simulink library "bcm"  (R2021b)
settings: Solver=VariableStepAuto  StartTime=0.0  StopTime=10.0  RelTol=1e-3
undefined symbols (not defined in the file or in its folder): ENUM_ANTITHEFT_ALARM, ENUM_ANTITHEFT_ARM, ENUM_ANTITHEFT_DISARM, ENUM_ANTITHEFT_WAIT, ENUM_GEARPOSNTOCAN_P, ENUM_PDKEYRAWLULOCK_INUNLOCK, ENUM_PDKEYRAWPS_INPS, ENUM_POWERSTA_READY, ENUM_POWERSTA_STANDBY, FALSE, KBCM_ALMBrightnessDark_enum, KBCM_AmbBlue_enum, KBCM_AmbBreathT_K, KBCM_AmbBreathTOut_K, KBCM_AmbGreen_enum, KBCM_AmbLightUser_enum, KBCM_AmbPreset_enum, KBCM_AmbRed_enum, KBCM_Antitheft_enum_ovrdflg, KBCM_Antitheft_enum_ovrdval, KBCM_APMDoorCtrlSta_flg_ovrdflg, KBCM_APMDoorCtrlSta_flg_ovrdval, KBCM_DelayTSW_flg, KBCM_DiagFLTC_mA, KBCM_DiagFMHT_s, KBCM_DiagFRTC_mA, KBCM_DiagRLTC_mA, KBCM_DiagRRTC_mA, KBCM_DrAPMRetryTimes_cnt, KBCM_DrOpenWdwOT_s, KBCM_DrOpenWdwReady_s, KBCM_ESSOffT_ms, KBCM_ESSOnT_ms, KBCM_IVIRstHoldT_ms, KBCM_IVIRstTriggerT_ms, KBCM_ONDelayT_ms, KBCM_ReDetectT_K, KBCM_RmLampKeep_min, KBCM_RmLpKeyInT_s, KBCM_RmLpKeyMissT_s, KBCM_SlpDebounceTime_s, KBCM_SPTGDetectT_sec, KBCM_SPTGLeave_flg, KBCM_SPTGLeftBound_cm, KBCM_SPTGLeftBoundOut_cm, KBCM_SPTGLowerBound_cm, KBCM_SPTGLowerBoundOut_cm, KBCM_SPTGRightBound_cm, KBCM_SPTGRightBoundOut_cm, KBCM_SPTGTOut_K, KBCM_SPTGUpperBound_cm, KBCM_SPTGUpperBoundOut_cm, KBCM_SPTGWaitDKC_sec, KBCM_USSDis_cm, KBCM_USSFilterT_K, KBCM_WaitAPMPwr_K, KBCM_WdwManualDetT_s, MIN2SEC, TRUE, XX2KXX
libraries: simulink x41, $bdroot x3, hcu_lib x2
(part 5 of 6)

== stateflow chart bcm/BCM/BCM/ExteriorLight/Chart ==
  settings: updateMethod=DISCRETE
  state FollowMeSW [parallel]
    settings: executionOrder=2
    state sRelease
    state sPress
    (default) -> sRelease
    sRelease -> sPress : [VINP_FollowMeSW_flg==1]/{AutoCut.eFollow;}
    sPress -> sRelease : [VINP_FollowMeSW_flg==0]
  state RFogLamp [parallel]
    settings: executionOrder=1
    state sON
      en:VBCM_RrFogLamp_flg=1;
    state sOFF
      en:VBCM_RrFogLamp_flg=0;
    (default) -> RFogLamp.sOFF
    RFogLamp.sOFF -> RFogLamp.sON : [VPMM_PwrSta_enum>3&&....
        | VINP_RFogLampSW_flg==1&&....
        | VBCM_LBeam_flg==1]
    RFogLamp.sON -> RFogLamp.sOFF : [VPMM_PwrSta_enum<=3||....
        | VINP_RFogLampSW_flg==0||....
        | VBCM_LBeam_flg==0]
  state DRL [parallel]
    settings: executionOrder=3
    state sOFF
      en:VBCM_LDRL_flg=0;
      VBCM_RDRL_flg=0;
    state DRL_Opearting
      state sDebounce
      state sON
        en:VBCM_LDRL_flg=1;
        VBCM_RDRL_flg=1;
      note: 300 ms
      state TurnLeft
        en:VBCM_LDRL_flg=0;
        VBCM_RDRL_flg=1;
      state TurnRight
        en:VBCM_LDRL_flg=1;
        VBCM_RDRL_flg=0;
      sDebounce -> (junction 2687) : [after(30,tick)]
      (junction 2687) -> DRL.DRL_Opearting.sON [order 1] : [VBCM_OutMode_enum==0]
      (junction 2687) -> (junction 2689) [order 2]
      DRL.DRL_Opearting.sON -> TurnLeft [order 1] : [VBCM_OutMode_enum==1]
      TurnLeft -> DRL.DRL_Opearting.sON [order 1] : [VBCM_OutMode_enum==0]
      TurnRight -> DRL.DRL_Opearting.sON [order 2] : [VBCM_OutMode_enum==0]
      DRL.DRL_Opearting.sON -> TurnRight [order 2] : [VBCM_OutMode_enum==2]
      (junction 2689) -> TurnLeft [order 1] : [VBCM_OutMode_enum==1]
      (junction 2689) -> (junction 2701) [order 2]
      TurnRight -> TurnLeft [order 1] : [VBCM_OutMode_enum==1]
      TurnLeft -> TurnRight [order 2] : [VBCM_OutMode_enum==2]
      (junction 2701) -> TurnRight
    (default) -> DRL.sOFF
    DRL.sOFF -> sDebounce : [VBCM_DiagDRLOFF_flg==0 &&...
        | VPMM_PwrSta_enum==ENUM_POWERSTA_READY &&...
        | (VTQD_ShiftGearPosn_enum != ENUM_GEARPOSNTOCAN_P || VINP_HeadLampSW_enum==0) &&...
        | !VBCM_PosLamp_flg &&...
        | VBCM_OutMode_enum < 3]
    DRL_Opearting -> DRL.sOFF : [VBCM_DiagDRLOFF_flg==1 ||...
        | VPMM_PwrSta_enum!=ENUM_POWERSTA_READY ||...
        | (VTQD_ShiftGearPosn_enum == ENUM_GEARPOSNTOCAN_P && VINP_HeadLampSW_enum!=0) ||...
        | VBCM_PosLamp_flg ||...
        | VBCM_OutMode_enum >= 3]
  state sBrakeLamp [parallel]
    settings: executionOrder=4
    state sON
      en:VBCM_BrakeLamp_flg=1;
    state sOFF
      en:VBCM_BrakeLamp_flg=0;
    (default) -> sBrakeLamp.sOFF
    sBrakeLamp.sOFF -> sBrakeLamp.sON : [VINP_BrakeSWGPIO_flg==1 || VTQD_ReBrakeLPReq_flg==1 || VINP_ActBrkLampSta_flg==1]
    sBrakeLamp.sON -> sBrakeLamp.sOFF : [VINP_BrakeSWGPIO_flg==0 && VTQD_ReBrakeLPReq_flg==0 && VINP_ActBrkLampSta_flg==0]
  state sReverseLamp [parallel]
    settings: executionOrder=5
    state sON
      en:VBCM_ReverseLamp_flg=1;
    state sOFF
      en:VBCM_ReverseLamp_flg=0;
    (default) -> sReverseLamp.sOFF
    sReverseLamp.sOFF -> sReverseLamp.sON : [VPMM_PwrSta_enum>3&&VTQD_ShiftGearPosn_enum==7]
    sReverseLamp.sON -> sReverseLamp.sOFF : [VPMM_PwrSta_enum<=3||VTQD_ShiftGearPosn_enum!=7]
  state sATCtrl [parallel]
    settings: executionOrder=6
    state StandBy
    state Lock
      en:send(AutoCut.eLock);
    state Unlock
      en:send(AutoCut.eUnlock);
    (default) -> StandBy
    StandBy -> Lock [order 1] : [VBCM_ATCtrl_enum==1]
    Lock -> StandBy : [VBCM_ATCtrl_enum!=1]
    StandBy -> sATCtrl.Unlock [order 2] : [VBCM_ATCtrl_enum==2]
    sATCtrl.Unlock -> StandBy : [VBCM_ATCtrl_enum!=2]
  state PositionLamp [parallel]
    settings: executionOrder=11
    state sPositionLamp
      en:VBCM_PosLamp_flg=1;
    state sOFF
      en:VBCM_PosLamp_flg=0;
    (default) -> PositionLamp.sOFF
    (junction 2636) -> sPositionLamp [order 1] : [VINP_HeadLampSW_enum==1||VINP_HeadLampSW_enum==2]
    PositionLamp.sOFF -> (junction 2636) [order 1] : [!VBCM_AutoCut_flg]
    (junction 2636) -> (junction 2637) [order 2]
    (junction 2637) -> sPositionLamp [order 1] : [VPMM_PwrSta_enum>3&&VINP_HeadLampSW_enum==0&&VINP_RLSLampSta_flg]
    (junction 2637) -> (junction 2638) [order 2]
    (junction 2638) -> sPositionLamp : [VBCM_FollowMe_flg]
    PositionLamp.sOFF -> sPositionLamp [order 2] : [VBCM_showup_flg]
    (junction 2639) -> PositionLamp.sOFF : [!VBCM_FollowMe_flg&&(VINP_HeadLampSW_enum==3||....
        | (VINP_HeadLampSW_enum==0&&(VPMM_PwrSta_enum<=3||!VINP_RLSLampSta_flg)))]
    (junction 2640) -> (junction 2639) [order 2]
    (junction 2640) -> PositionLamp.sOFF [order 1] : [VBCM_AutoCut_flg]
    sPositionLamp -> (junction 2640) : [!VBCM_showup_flg]
  state AutoCut [parallel]
    settings: executionOrder=12
    state FollowMeHome
      en:
      VBCM_FollowMe_flg=1;
      VBCM_AutoCut_flg=0;
      VBCM_showup_flg=0;
      ex:
      VBCM_FollowMe_flg=0;
    state Normal
      state sNormal
        en:VBCM_AutoCut_flg=0;
        VBCM_showup_flg=0;
      state AutoCutDetect
      note: 40 sec
      state Unlock
        en:VBCM_AutoCut_flg=1;
        VBCM_showup_flg=1;
        note: 30 sec
      state AutoCut
        en:VBCM_AutoCut_flg=1;
        VBCM_showup_flg=0;
        VBCM_FollowMe_flg=0;
      sNormal -> AutoCutDetect : [VPMM_PwrSta_enum<=3&&(VINP_HeadLampSW_enum!=3)]
      (junction 2665) -> sNormal : [VPMM_PwrSta_enum>3||VINP_HeadLampSW_enum==3]
      AutoCutDetect -> (junction 2665) [order 1]
      AutoCut.Normal.AutoCut -> (junction 2665)
      AutoCutDetect -> AutoCut.Normal.AutoCut [order 2] : eLock
      AutoCutDetect -> AutoCut.Normal.AutoCut [order 3] : [after(4000,tick)]
      AutoCut.Normal.Unlock -> sNormal [order 2] : [VPMM_PwrSta_enum>3]
      (default) -> AutoCut.Normal.AutoCut
      AutoCut.Normal.Unlock -> AutoCut.Normal.AutoCut [order 1] : eLock
      AutoCut.Normal.Unlock -> AutoCut.Normal.AutoCut [order 3] : [after(3000,tick)]
      Normal -> AutoCut.Normal.Unlock [order 1] : eUnlock[VPMM_PwrSta_enum<=3]
    note: 4000
    note: 40 sec
    (default) -> Normal
    Normal -> FollowMeHome [order 1] : eFollow[VPMM_PwrSta_enum<=3]
    FollowMeHome -> sNormal [order 2] : eFollow
    FollowMeHome -> sNormal [order 3] : [VPMM_PwrSta_enum>3]
    FollowMeHome -> (junction 2717) [order 1] : [after(VBCM_DiagFMHT_s,tick)]
    (junction 2717) -> sNormal [order 1] : [VPMM_PwrSta_enum>3||...
        |  VINP_HeadLampSW_enum==3]
    (junction 2717) -> (junction 2719) [order 2]
    (junction 2719) -> AutoCut.Normal.AutoCut
  state LowBeam [parallel]
    settings: executionOrder=8
    state sLBeam
      en:VBCM_LBeam_flg=1;
    state sOFF
      en:VBCM_LBeam_flg=0;
    (default) -> LowBeam.sOFF
    (junction 2417) -> sLBeam [order 1] : [VBCM_HBeam_flg]
    LowBeam.sOFF -> (junction 2417) [order 1] : [!VBCM_AutoCut_flg]
    (junction 2417) -> (junction 2418) [order 2]
    (junction 2418) -> sLBeam [order 1] : [VINP_HeadLampSW_enum==2]
    (junction 2418) -> (junction 2419) [order 2]
    (junction 2419) -> sLBeam [order 1] : [VPMM_PwrSta_enum>3&&VINP_HeadLampSW_enum==0&&VINP_RLSLampSta_flg]
    (junction 2419) -> (junction 2420) [order 2]
    (junction 2420) -> sLBeam : [VBCM_FollowMe_flg]
    LowBeam.sOFF -> sLBeam [order 2] : [VBCM_showup_flg]
    (junction 2421) -> LowBeam.sOFF [order 1] : [VBCM_AutoCut_flg]
    sLBeam -> (junction 2421) : [!VBCM_showup_flg]
    (junction 2421) -> (junction 2422) [order 2]
    (junction 2422) -> LowBeam.sOFF : [!VBCM_FollowMe_flg&&!VBCM_HBeam_flg&&VINP_HeadLampSW_enum!=2&&....
        | (VINP_HeadLampSW_enum!=0||!VINP_RLSLampSta_flg||VPMM_PwrSta_enum<=3)]
  state HighBeam [parallel]
    settings: executionOrder=7
    state sHBeam
      en:VBCM_HBeam_flg=1;
    state sOFF
      en:VBCM_HBeam_flg=0;
    (default) -> HighBeam.sOFF
    HighBeam.sOFF -> (junction 2455) : [!VBCM_AutoCut_flg]
    (junction 2455) -> sHBeam [order 1] : [VINP_CSWPassSWSta_flg]
    (junction 2455) -> (junction 2456) [order 2]
    (junction 2456) -> (junction 2457) : [VINP_CSWDimSw_flg]
    (junction 2457) -> sHBeam [order 1] : [VINP_HeadLampSW_enum==2]
    (junction 2457) -> (junction 2458) [order 2]
    (junction 2458) -> sHBeam : [VINP_HeadLampSW_enum==0&&VINP_RLSLampSta_flg==1&&VINP_ForceLowBeam_enum==0&&VPMM_PwrSta_enum>3&&VBCM_AutoHLB_flg]
    sHBeam -> HighBeam.sOFF [order 1] : [VBCM_AutoCut_flg]
    (junction 2459) -> HighBeam.sOFF [order 1] : [!VINP_CSWDimSw_flg]
    sHBeam -> (junction 2459) [order 2] : [!VINP_CSWPassSWSta_flg]
    (junction 2459) -> (junction 2605) [order 2]
    (junction 2460) -> HighBeam.sOFF [order 1] : [VINP_HeadLampSW_enum!=0]
    (junction 2605) -> (junction 2460) : [VINP_HeadLampSW_enum!=2]
    (junction 2460) -> (junction 2462) [order 2]
    (junction 2462) -> HighBeam.sOFF [order 1] : [VINP_RLSLampSta_flg==0||VPMM_PwrSta_enum<=3]
    (junction 2462) -> (junction 2463) [order 2]
    (junction 2463) -> HighBeam.sOFF : [VINP_ForceLowBeam_enum==1||!VBCM_AutoHLB_flg]
  state AutoHLB [parallel]
    settings: executionOrder=13
    state AutoON
      on after(KBCM_ONDelayT_ms, tick):
      VBCM_AutoHLB_flg = TRUE;
    state AutoOFF
      en:
      VBCM_AutoHLB_flg = FALSE;
    (default) -> AutoOFF
    AutoOFF -> AutoON : [VINP_METERKPHCalcu_kph >= 30]
    AutoON -> AutoOFF : [VINP_METERKPHCalcu_kph <= 25]
  state RBSD_CTRL [parallel]
    settings: executionOrder=10
    state OFF
      en:VBCM_RBSD_flg=0;
    state FlashOFF
      en:VBCM_RBSD_flg=0;
    state ON
      en:VBCM_RBSD_flg=1;
    (default) -> RBSD_CTRL.OFF
    RBSD_CTRL.FlashOFF -> RBSD_CTRL.OFF [order 1] : [VINP_SRRBSDWarnR_flg==0 && VINP_SRRODAWarnR_flg==0]
    RBSD_CTRL.ON -> RBSD_CTRL.FlashOFF [order 2] : [after(13,tick)&&(VINP_SRRBSDWarnR_flg==2||VINP_SRRODAWarnR_flg==2)]
    RBSD_CTRL.FlashOFF -> RBSD_CTRL.ON [order 2] : [after(12,tick)]
    RBSD_CTRL.ON -> RBSD_CTRL.OFF [order 1] : [VINP_SRRBSDWarnR_flg==0 && VINP_SRRODAWarnR_flg==0]
    RBSD_CTRL.OFF -> RBSD_CTRL.ON : [VINP_SRRBSDWarnR_flg>0 || VINP_SRRODAWarnR_flg>0]
  state LBSD_CTRL [parallel]
    settings: executionOrder=9
    state OFF
      en:VBCM_LBSD_flg=0;
    state FlashOFF
      en:VBCM_LBSD_flg=0;
    state ON
      en:VBCM_LBSD_flg=1;
    (default) -> LBSD_CTRL.OFF
    LBSD_CTRL.FlashOFF -> LBSD_CTRL.OFF [order 1] : [VINP_SRRBSDWarnL_flg==0 && VINP_SRRODAWarnL_flg==0]
    LBSD_CTRL.ON -> LBSD_CTRL.FlashOFF [order 2] : [after(13,tick)&&(VINP_SRRBSDWarnL_flg==2||VINP_SRRODAWarnL_flg==2)]
    LBSD_CTRL.FlashOFF -> LBSD_CTRL.ON [order 2] : [after(12,tick)]
    LBSD_CTRL.ON -> LBSD_CTRL.OFF [order 1] : [VINP_SRRBSDWarnL_flg==0 && VINP_SRRODAWarnL_flg==0]
    LBSD_CTRL.OFF -> LBSD_CTRL.ON : [VINP_SRRBSDWarnL_flg>0 || VINP_SRRODAWarnL_flg>0]
  data: VPMM_PwrSta_enum input uint8 [0..5]; VINP_HeadLampSW_enum input uint8 [0..3]; VINP_RFogLampSW_flg input boolean; VINP_BrakeSWGPIO_flg input boolean; VINP_CSWDimSw_flg input boolean; VINP_CSWPassSWSta_flg input boolean; VTQD_ShiftGearPosn_enum input uint8 [0..15]; VBCM_PosLamp_flg output boolean; VBCM_LBeam_flg output boolean; VBCM_HBeam_flg output boolean; VBCM_RrFogLamp_flg output boolean; VBCM_BrakeLamp_flg output boolean; VBCM_ReverseLamp_flg output boolean; VBCM_OutMode_enum input uint8 [0..15]; VBCM_AutoCut_flg local boolean; VBCM_LDRL_flg output boolean; VBCM_RDRL_flg output boolean; VINP_FollowMeSW_flg input boolean; VBCM_ATCtrl_enum input uint8 [0..2]; VINP_RLSLampSta_flg input boolean; VINP_ActBrkLampSta_flg input boolean; VINP_SRRODAWarnR_flg input; VINP_SRRODAWarnL_flg input; VINP_SRRBSDWarnR_flg input; VINP_SRRBSDWarnL_flg input; VINP_ForceLowBeam_enum input uint8; VTQD_ReBrakeLPReq_flg input; VBCM_LBSD_flg output boolean; VBCM_RBSD_flg output boolean; VBCM_DiagDRLOFF_flg input; VBCM_DiagFMHT_s input; ENUM_GEARPOSNTOCAN_P parameter; ENUM_POWERSTA_READY parameter; VBCM_showup_flg output boolean; VBCM_AutoHLB_flg local boolean =0; VINP_METERKPHCalcu_kph input; KBCM_ONDelayT_ms input; VBCM_FollowMe_flg output boolean; TRUE parameter; FALSE parameter
  events: eLock local FUNCTION_CALL_EVENT; eUnlock local FUNCTION_CALL_EVENT; eFollow local FUNCTION_CALL_EVENT

== stateflow chart bcm/BCM/BCM/FlasherSignal/Chart ==
  settings: updateMethod=DISCRETE
  state sModeSelect [parallel]
    settings: executionOrder=2  description=This state models the modes of a door sensor and implements logic to respond when that sensor is producing a signal.
    state sStandBy
    (default) -> sStandBy
      settings: description=On the first sample call the door mode is set to active.
    sStandBy -> (junction 1892)
    (junction 1893) -> sStandBy
    (junction 1892) -> (junction 1893) [order 1] : [ATAlarm==1]{InputMode=6;}
    (junction 1892) -> (junction 1969) [order 2]
    (junction 1971) -> (junction 1893)
    (junction 1969) -> (junction 1971) [order 1] : [InputMode==4||InputMode==5||InputMode==9]
    (junction 1969) -> (junction 2027) [order 2]
    (junction 2028) -> (junction 1971)
    (junction 2027) -> (junction 2028) [order 1] : [SPTGDet==1]{InputMode=8;}
    (junction 2027) -> (junction 1871) [order 2]
    (junction 1873) -> (junction 2028)
    (junction 1871) -> (junction 1873) [order 1] : [PwrSta>3&&ESS_Active==1]{InputMode=7;}
    (junction 1871) -> (junction 1987) [order 2]
    (junction 1989) -> (junction 1873)
    (junction 1987) -> (junction 1989) [order 1] : [HazardSW==1 || VBCM_PwrErrWarn_flg]{InputMode=3;}
    (junction 1987) -> (junction 1876) [order 2]
    (junction 1878) -> (junction 1989)
    (junction 1876) -> (junction 1878) [order 1] : [PwrSta>3&&CSW_TurnSw_Sta==1]{InputMode=1;}
    (junction 1876) -> (junction 1882) [order 2]
    (junction 1884) -> (junction 1878)
    (junction 1882) -> (junction 1884) [order 1] : [PwrSta>3&&CSW_TurnSw_Sta==2]{InputMode=2;}
    (junction 1882) -> (junction 2013) [order 2]
    (junction 2014) -> (junction 1884)
    (junction 2013) -> (junction 2014) [order 1] : [PwrSta>3&&(LeftTurnLightReq==1||APS_LTurnReq==1)]{InputMode=1;}
    (junction 2013) -> (junction 2007) [order 2]
    (junction 2009) -> (junction 2014)
    (junction 2007) -> (junction 2009) [order 1] : [PwrSta>3&&(RightTurnLightReq==1||APS_RTurnReq==1)]{InputMode=2;}
    (junction 2007) -> (junction 1887) [order 2]
    (junction 1889) -> (junction 2009)
    (junction 1887) -> (junction 1889) : /{InputMode=0;}
  state sPTGReq [parallel]
    settings: executionOrder=5
    state StandBy
    state Twice
      en:InputMode=9;
    state ThreeTimes
      en:InputMode=5;
    (default) -> sPTGReq.StandBy
    sPTGReq.StandBy -> Twice [order 1] : [PTG_RDIL_Sta==1]
    Twice -> sPTGReq.StandBy : [PTG_RDIL_Sta==0]
    sPTGReq.StandBy -> ThreeTimes [order 2] : [PTG_RDIL_Sta==2]
    ThreeTimes -> sPTGReq.StandBy : [PTG_RDIL_Sta==0]
  state HazardSW [parallel]
    settings: executionOrder=1
    state Normal
      state sHAZARDOFF
      state Press
      state sHAZARDON
      (default) -> sHAZARDOFF
      sHAZARDOFF -> Press : [HazardSWSta==1]/{HazardSW=1;}
      (junction 1864) -> sHAZARDOFF [order 1] : [HazardSW==0]
      Press -> (junction 1864) : [HazardSWSta==0]
      (junction 1864) -> sHAZARDON [order 2]
      sHAZARDON -> Press : [HazardSWSta==1]{HazardSW=0;}
    state ADASHazardReq
    (default) -> Normal
    ADASHazardReq -> sHAZARDON : [HazardWarningReq==0]
    Normal -> ADASHazardReq : [HazardWarningReq==1]{HazardSW=1}
  state sATCtrl [parallel]
    settings: executionOrder=4
    state StandBy
    state Lock
      en:InputMode=4;
    state Unlock
      en:InputMode=5;
    (default) -> sATCtrl.StandBy
    sATCtrl.StandBy -> Lock [order 1] : [ATCtrl==1]
    Lock -> sATCtrl.StandBy : [ATCtrl!=1]
    sATCtrl.StandBy -> Unlock [order 2] : [ATCtrl==2]
    Unlock -> sATCtrl.StandBy : [ATCtrl!=2]
  state sPowerErrorWarning [parallel]
    settings: executionOrder=6
    state sWarningOFF
      en:
      VBCM_PwrErrWarn_flg = FALSE;
    state sWarningON
      en:
      VBCM_PwrErrWarn_flg = TRUE;
    (default) -> sWarningOFF
    sWarningOFF -> sWarningON : [PwrSta == ENUM_POWERSTA_STANDBY && ...
        |  (VDDM_HVRlyOpCFS_flg || VDDM_MCUActCFS_flg)]
    sWarningON -> sWarningOFF : [PwrSta != ENUM_POWERSTA_STANDBY || ...
        |  (!VDDM_HVRlyOpCFS_flg && !VDDM_MCUActCFS_flg)]
  state Main [parallel]
    settings: executionOrder=3
    state sUnLockOFF1
      en:InputMode=0;
    state sUnLockOFF
      en:LTurnLP=0;
      RTurnLP=0;
      FlashCount=FlashCount-1;
    state sHazardOFF
      en:LTurnLP=0;
      RTurnLP=0;
    state sESSOFF
      en:LTurnLP=0;
      RTurnLP=0;
    state sLockOFF
      en:LTurnLP=0;
      RTurnLP=0;
      InputMode=0;
    state sAlarmOFF
      en:LTurnLP=0;
      RTurnLP=0;
    note: 500 ms
    note: 600 ms
    note: 500 ms
    note: 460 ms
    note: 460 ms
    note: 200 ms
    note: 100 ms
    state sHazardON
      en:LTurnLP=1;
      RTurnLP=1;
    state sESSON
      en:LTurnLP=1;
      RTurnLP=1;
    state sLock
      en:LTurnLP=1;
      RTurnLP=1;
    state sAlarm
      en:LTurnLP=1;
      RTurnLP=1;
    state sUnlock
      en:LTurnLP=1;
      RTurnLP=1;
    state sWait
      en:LTurnLP=0;RTurnLP=0;
    note: 120 ms
    state sOFF
      en:LTurnLP=0;RTurnLP=0;
    state sLeftON
      en:LTurnLP=1;
      RTurnLP=0;
    state sRightON
      en:LTurnLP=0;
      RTurnLP=1;
    state sSPTG
      en:LTurnLP=1;
      RTurnLP=1;
      BCMBuzzerReq=1;
      ex:
      BCMBuzzerReq=0;
    note: 230 ms
    note: 230 ms
    state sOFFNG
      en:LTurnLP=0;
      RTurnLP=0;
    note: 500 ms
    note: 500 ms
    state sSPTGOFF
      en:LTurnLP=0;
      RTurnLP=0;
      BCMBuzzerReq=0;
    note: 230 ms
    note: 230 ms
    state sRightKeep
    state sLeftKeep
    note: 230 ms
    state sOFFOK
      en:LTurnLP=0;
      RTurnLP=0;
    Main -> sWait : [OutMode!=InputMode]
        | {OutMode=InputMode;}
    sUnLockOFF -> sUnLockOFF1 [order 1] : [FlashCount==0]
    sLock -> sLockOFF : [after(50,tick)]
    sAlarm -> sAlarmOFF : [after(50,tick)]
    sAlarmOFF -> sAlarm : [after(50,tick)]
    sHazardON -> sHazardOFF : [after(46,tick)]
    sHazardOFF -> sHazardON : [after(46,tick)]
    sESSON -> sESSOFF : [after(VBCM_ESSOnT_tick,tick)]
    sESSOFF -> sESSON : [after(VBCM_ESSOffT_tick,tick)]
    sUnlock -> sUnLockOFF : [after(20,tick)]
    sUnLockOFF -> sUnlock [order 2] : [after(60,tick)]
    sOFF -> sUnlock [order 9] : [InputMode==9]....
        | {FlashCount=2;}
    sOFF -> sUnlock [order 4] : [OutMode==5]....
        | {FlashCount=3;}
    sOFF -> sLock [order 1] : [OutMode==4]
    sOFF -> sAlarm [order 5] : [OutMode==6]
    sOFF -> sHazardON [order 8] : [OutMode==3]
    sOFF -> sESSON [order 3] : [OutMode==7]
    (default) -> sOFF
    sWait -> sOFF : [after(12,tick)]
    sOFF -> sSPTG [order 2] : [OutMode==8]
    sOFF -> sLeftON [order 6] : [OutMode==1]
    sOFF -> sRightON [order 7] : [OutMode==2]
    (junction 1940) -> sLeftON [order 1] : [OutMode==1]
    (junction 1940) -> sRightON [order 2]
    sOFFNG -> (junction 1940) : [after(23,tick)]
    sLeftON -> (junction 1918) : [after(23,tick)]
    sRightON -> (junction 1929) : [after(23,tick)]
    sSPTG -> sSPTGOFF : [after(50,tick)]
    sSPTGOFF -> sSPTG : [after(50,tick)]
    (junction 2062) -> sOFFNG [order 1] : [FRTurnLampC>DiagFRTC]
        | {DiagFRTS=0;DiagRRTS=1;}
    (junction 1929) -> (junction 2062) [order 2]
    (junction 1918) -> (junction 2053) [order 2]
    (junction 2053) -> sOFFNG [order 1] : [FLTurnLampC>DiagFLTC]
        | {DiagFLTS=0;DiagRLTS=1;}
    (junction 2062) -> (junction 2065) [order 2]
    (junction 1929) -> sRightKeep [order 1] : [RRTurnLampC>DiagRRTC &&...
        | FRTurnLampC>DiagFRTC]
        | {DiagFRTS=0;DiagRRTS=0;}
    (junction 1918) -> sLeftKeep [order 1] : [RLTurnLampC>DiagRLTC &&...
        | FLTurnLampC>DiagFLTC]
        | {DiagFLTS=0;DiagRLTS=0;}
    (junction 2053) -> (junction 2056) [order 2]
    (junction 2056) -> sOFFNG [order 1] : [RLTurnLampC>DiagRLTC]
        | {DiagFLTS=1;DiagRLTS=0;}
    (junction 2065) -> sOFFNG [order 1] : [RRTurnLampC>DiagRRTC]
        | {DiagFRTS=1;DiagRRTS=0;}
    (junction 2056) -> (junction 2059) [order 2]
    (junction 2065) -> (junction 2068) [order 2]
    (junction 2059) -> sOFFNG : {DiagFLTS=1;DiagRLTS=1;}
    (junction 2068) -> sOFFNG : {DiagFRTS=1;DiagRRTS=1;}
    sOFFOK -> sOFFNG : [after(23,tick)]
    sRightKeep -> sOFFOK : [after(23,tick)]
    sLeftKeep -> sOFFOK : [after(23,tick)]
  data: ATCtrl input uint8 [0..2]; ATAlarm input boolean; PwrSta input uint8 [0..5]; HazardSWSta input boolean [0..1]; CSW_TurnSw_Sta input uint8 [0..3]; RLTurnLampC input [0..255]; RRTurnLampC input [0..255]; FLTurnLampC input [0..255]; FRTurnLampC input [0..255]; PTG_RDIL_Sta input; HazardSW output boolean =0; LTurnLP output boolean; RTurnLP output boolean; InputMode local uint8; FlashCount local uint8; OutMode output uint8; ESS_Active input boolean; LeftTurnLightReq input boolean; RightTurnLightReq input boolean; SPTGDet input boolean; HazardWarningReq input; DiagFLTC input; DiagFRTC input; DiagRLTC input; DiagRRTC input; APS_LTurnReq input; APS_RTurnReq input; DiagFLTS output; DiagFRTS output; DiagRLTS output; DiagRRTS output; BCMBuzzerReq output boolean; FALSE parameter; TRUE parameter; ENUM_POWERSTA_STANDBY parameter; VDDM_HVRlyOpCFS_flg input; VDDM_MCUActCFS_flg input; VBCM_PwrErrWarn_flg local boolean; VBCM_ESSOffT_tick input; VBCM_ESSOnT_tick input

== stateflow chart bcm/BCM/BCM/PowerMirror/Chart ==
  settings: sampleTime=StepSize
  state sPowerFlag [parallel]
    settings: executionOrder=1
    state sActive
      en:PFlag=1;
    state sOff
      en:PFlag=0;
    state sDelay
      en:PFlag=1;
    (default) -> sOff
    sOff -> sActive : [PwrSta>3]
    sDelay -> sActive [order 1] : [PwrSta>3]
    sActive -> sDelay : [PwrSta<=3]
    (junction 1609) -> sOff
    sDelay -> (junction 1609) [order 2] : [after(3000,tick)]
  state sMirrorFoldSw [parallel]
    settings: executionOrder=2  description=This state models the modes of a door sensor and implements logic to respond when that sensor is producing a signal.
    state sRelease
    state sPush
      en:sMain.eMFSW;
    (default) -> sRelease
      settings: description=On the first sample call the door mode is set to active.
    sPush -> sRelease : [!MirrorFoldSw]
    sRelease -> sPush : [MirrorFoldSw]
  state sMain [parallel]
    settings: executionOrder=5
    state Close
      en:MirrorCtrl=0;
      MirrorFlodPos=0;
    state Mirror2Open
      en:MirrorCtrl=2;
    state Suspend2Open
      en:MirrorCtrl=0;
    state Suspend2Close
      en:MirrorCtrl=0;
    state Mirror2Close
      en:MirrorCtrl=1;
    state Open
      en:MirrorCtrl=0;MirrorFlodPos=1;
    (default) -> (junction 1695) : {MFSWTri=EEP_MFSWTri_flg;}
    (junction 1695) -> (junction 1697) [order 2]
    (junction 1695) -> Close [order 1] : [!EEP_MirrorFlodPos]{DisAntiTheftReq=EEP_MFSWTri_flg;}
    (junction 1697) -> Open
    Close -> (junction 1669) [order 1] : eMirrorUnlock[PwrSta<=4&&!DisAntiTheftReq]
    (junction 1669) -> (junction 1670)
    Close -> (junction 1670) [order 2] : eMFSW[PFlag]/{DisAntiTheftReq=0;}
    (junction 1670) -> (junction 1668)
    Close -> (junction 1668) [order 3] : eAutoOpen/{DisAntiTheftReq=0;}
    (junction 1668) -> Mirror2Open
    Suspend2Open -> (junction 1668) : [after(10,tick)]
    Mirror2Close -> Close [order 2] : [after(600,tick)]/{DisAntiTheftReq=MFSWTri;}
    Mirror2Open -> Suspend2Close [order 1] : eMirrorLock[PwrSta<=4]/{MFSWTri=0;}
    Mirror2Open -> Suspend2Close [order 2] : eMFSW[PFlag]/{MFSWTri=1}
    Mirror2Open -> Open [order 3] : [after(600,tick)]
    Mirror2Close -> Suspend2Open [order 1] : eMirrorUnlock[PwrSta<=4]
    Mirror2Close -> Suspend2Open [order 3] : eMFSW[PFlag]
    Suspend2Close -> (junction 1650) : [after(10,tick)]
    Open -> (junction 1650) [order 2] : eMFSW[PFlag]/{MFSWTri=1}
    (junction 1650) -> Mirror2Close
    (junction 1649) -> (junction 1650)
    Open -> (junction 1649) [order 1] : eMirrorLock[PwrSta<=4]/{MFSWTri=0;}
  state sATCtrl [parallel]
    settings: executionOrder=4
    state StandBy
    state Lock
      en: sMain.eMirrorLock;
    state Unlock
      en: sMain.eMirrorUnlock;
    (default) -> StandBy
    StandBy -> Lock [order 1] : [ATActCtrl==1]
    Lock -> StandBy : [ATActCtrl!=1]
    StandBy -> Unlock [order 2] : [ATActCtrl==2]
    Unlock -> StandBy : [ATActCtrl!=2]
  state sRemoteControl [parallel]
    settings: executionOrder=6
    state Standby
    state Fold
      en: sMain.eMirrorLock;
    state Unfold
      en: sMain.eMirrorUnlock;
    (default) -> Standby
    Standby -> Fold [order 1] : [VINP_ReOutsideMirror_enum == 1]
    Fold -> Standby : [VINP_ReOutsideMirror_enum != 1]
    Standby -> Unfold [order 2] : [VINP_ReOutsideMirror_enum == 2]
    Unfold -> Standby : [VINP_ReOutsideMirror_enum != 2]
  state sAutoOpen [parallel]
    settings: executionOrder=3
    state Reset
    state AutoOpenRequest
      en:sMain.eAutoOpen;
    (default) -> Reset
    Reset -> AutoOpenRequest : [VehSpeed>30 &&...
        | VehSpeed<256 &&...
        | PwrSta>3]
    AutoOpenRequest -> Reset : [PwrSta<=3]
  data: PwrSta input uint8 [0..4]; MirrorFoldSw input boolean; VehSpeed input [0..4096]; MirrorCtrl output uint8 [0..2] =0; PFlag local boolean; DisAntiTheftReq local boolean =0; ATActCtrl input uint8 [0..2]; VINP_ReOutsideMirror_enum input; MFSWTri output boolean =0; EEP_MFSWTri_flg input; MirrorFlodPos output; EEP_MirrorFlodPos input
  data VehSpeed settings: description=Min=0, Max=2047, Engineering Unit = km/h, Offset=0 km/h, Resolution= 0.125 km/h per bit, >2047 = Invalid (bit 12 = 1)
  data MirrorCtrl settings: description=|
      | Bcm Buzzer output results.
      | 0 = None Buzzer
      | 1 = Turn signal Buzzer
      | 2 = Key Reminder Buzzer
      | 3 = Seat Belt Buzzer
      | 4 = Light Monitor Buzzer
  events: eAutoOpen local EITHER_EDGE_EVENT; eMFSW local EITHER_EDGE_EVENT; eMirrorUnlock local FUNCTION_CALL_EVENT; eMirrorLock local FUNCTION_CALL_EVENT

== stateflow chart bcm/BCM/BCM/RearDefogger/Chart ==
  settings: sampleTime=StepSize
  state CANCMD [parallel]
    settings: executionOrder=1
    state OFF
    state StandBy
    state Press
    (default) -> OFF
    OFF -> StandBy : [PwrSta>3]
    StandBy -> OFF [order 1] : [PwrSta<=3]
    StandBy -> Press [order 2] : [RR_Def_Sta||IVI_RR_Def_Req]{sMain.eRRDefPress;}
    Press -> StandBy [order 2] : [!RR_Def_Sta&&!IVI_RR_Def_Req]
    Press -> OFF [order 1] : [PwrSta<=3]
  state sMain [parallel]
    settings: executionOrder=2  description=This state models the modes of a door sensor and implements logic to respond when that sensor is producing a signal.
    state sOFF
      en:MirrorDefog=0;
      RearDefog=0;
    state sON
      en:MirrorDefog=1;
      RearDefog=1;
    note: 20 min
    (default) -> sOFF
      settings: description=On the first sample call the door mode is set to active.
    sOFF -> sON : eRRDefPress
    sON -> sOFF [order 1] : [PwrSta<=3]
    sON -> sOFF [order 2] : [after(120000,tick)]
    sON -> sOFF [order 3] : eRRDefPress
  data: PwrSta input uint8 [0..4]; RR_Def_Sta input boolean; IVI_RR_Def_Req input boolean; MirrorDefog output boolean =0; RearDefog output boolean
  data IVI_RR_Def_Req settings: description=Min=0, Max=2047, Engineering Unit = km/h, Offset=0 km/h, Resolution= 0.125 km/h per bit, >2047 = Invalid (bit 12 = 1)
  data MirrorDefog settings: description=|
      | Bcm Buzzer output results.
      | 0 = None Buzzer
      | 1 = Turn signal Buzzer
      | 2 = Key Reminder Buzzer
      | 3 = Seat Belt Buzzer
      | 4 = Light Monitor Buzzer
  events: eRRDefPress local FUNCTION_CALL_EVENT

== stateflow chart bcm/BCM/BCM/RoomLamp/Chart ==
  settings: sampleTime=StepSize
  state sDoorLockSta [parallel]
    settings: executionOrder=1  description=This state models the modes of a door sensor and implements logic to respond when that sensor is producing a signal.
    state sLock
    state sUnlock
    (default) -> (junction 1595)
    (junction 1595) -> sUnlock [order 2]
    (junction 1595) -> sLock [order 1] : [DrLockSW]
    sLock -> sUnlock : [DrLockSW==0]/sMain.eDrDoorUnlock
    sUnlock -> sLock : [DrLockSW==1]/sMain.eDrDoorLock
  state sRoomLampPower [parallel]
    settings: executionOrder=2
    state sON
      note: 40min
      state Keep
        en:
        RoomLampH=1;
        RoomLampTmr=0;
      state KeyIn
        en:
        RoomLampTmr=RoomLampTmr+task_time_s;
        du:
        RoomLampTmr=RoomLampTmr+task_time_s;
      state KeyMiss
        en:
        RoomLampTmr=RoomLampTmr+task_time_s;
        du:
        RoomLampTmr=RoomLampTmr+task_time_s;
      note: 10min
      (default) -> Keep
      Keep -> KeyIn [order 1] : [P_DKey_Area_LockUnlock==ENUM_PDKEYRAWLULOCK_INUNLOCK && ...
          |  P_DKey_Area_PS != ENUM_PDKEYRAWPS_INPS && ...
          |  PwrSta<4]
      KeyIn -> (junction 1756) [order 1] : [RoomLampTmr>=KBCM_RmLpKeyInT_s]
      (junction 1756) -> (junction 1760)
      KeyIn -> Keep [order 2] : [DoorOpen || PwrSta>3 || ...
          |  P_DKey_Area_PS==ENUM_PDKEYRAWPS_INPS]
      KeyMiss -> KeyIn [order 3] : [P_DKey_Area_LockUnlock==ENUM_PDKEYRAWLULOCK_INUNLOCK]
      KeyIn -> KeyMiss [order 3] : [P_DKey_Area_LockUnlock!=ENUM_PDKEYRAWLULOCK_INUNLOCK]
      KeyMiss -> Keep [order 2] : [DoorOpen || PwrSta>3 || ...
          |  P_DKey_Area_PS==ENUM_PDKEYRAWPS_INPS]
      KeyMiss -> (junction 1760) [order 1] : [RoomLampTmr>=KBCM_RmLpKeyMissT_s]
      Keep -> KeyMiss [order 2] : [P_DKey_Area_LockUnlock!=ENUM_PDKEYRAWLULOCK_INUNLOCK && ...
          |  P_DKey_Area_PS!=ENUM_PDKEYRAWPS_INPS && ...
          |  PwrSta<4]
    state sKeyON
      state sOFF
        en:RoomLampH=0;
      state sSAVEPower
        en:RoomLampH=0;
      state sKeep
        en:RoomLampH=1;
      sKeep -> sRoomLampPower.sKeyON.sOFF [order 2] : [AntitheftSta==1||AntitheftSta==3]
      sSAVEPower -> sRoomLampPower.sKeyON.sOFF : [AntitheftSta==1||AntitheftSta==3]
      (default) -> sSAVEPower
      sKeep -> sSAVEPower [order 1] : [after(KBCM_RmLampKeep_min,tick)]
    (default) -> sKeyON
    sRoomLampPower.sKeyON.sOFF -> sRoomLampPower.sON : [AntitheftSta==0||AntitheftSta==2]
    sKeyON -> sRoomLampPower.sON : [PwrSta>3||DoorOpen]
    sRoomLampPower.sON -> sKeep : [PwrSta<4&&!AllDoorSW&&!TailgateSW]
    (junction 1760) -> sSAVEPower
  state sMain [parallel]
    settings: executionOrder=3
    state sFunctionOFF
      en:RoomLampL=0;
    state sLampOFF
      state sOFF
        en:RoomLampL=0;
      state sKEEP
        en:RoomLampL=1;
      (junction 1665) -> sMain.sLampOFF.sOFF : [after(3000,tick)||PwrSta>=3]
      (junction 1666) -> sMain.sLampOFF.sOFF [order 2] : eDrDoorLock
      sMain.sLampOFF.sOFF -> sKEEP : eDrDoorUnlock[PwrSta<3]
      (junction 1666) -> (junction 1665) [order 1]
      sKEEP -> (junction 1666)
    state sON
      en:RoomLampL=1;
    (default) -> sFunctionOFF
    sFunctionOFF -> sMain.sLampOFF.sOFF : [RoomLampMode==0]
    sLampOFF -> sFunctionOFF [order 1] : [RoomLampMode==1]
    sMain.sON -> sFunctionOFF [order 1] : [RoomLampMode==1]
    (junction 1653) -> sMain.sLampOFF.sOFF
    (junction 1652) -> sKEEP [order 2]
    sLampOFF -> sMain.sON [order 2] : [AllDoorSW]
    (junction 1652) -> (junction 1653) [order 1] : [PwrSta>=3]
    sMain.sON -> (junction 1652) [order 2] : [AllDoorSW==0]
  data: task_time_s input single; PwrSta input uint8 [0..5]; RoomLampH output boolean =0; DrLockSW input boolean; AllDoorSW input boolean; DoorOpen input boolean; RoomLampL output boolean =0; AntitheftSta input uint8 [0..3]; TailgateSW input boolean; KBCM_RmLampKeep_min input; RoomLampMode input boolean =0; RoomLampTmr output single =0; P_DKey_Area_LockUnlock input uint8; P_DKey_Area_PS input uint8; KBCM_RmLpKeyInT_s input; KBCM_RmLpKeyMissT_s input; ENUM_PDKEYRAWPS_INPS parameter; ENUM_PDKEYRAWLULOCK_INUNLOCK parameter
  data RoomLampH settings: description=|
      | Bcm Buzzer output results.
      | 0 = None Buzzer
      | 1 = Turn signal Buzzer
      | 2 = Key Reminder Buzzer
      | 3 = Seat Belt Buzzer
      | 4 = Light Monitor Buzzer
  data DrLockSW settings: description=|
      | Door Lock Status
      | Lock =1
      | Unlock=0
  data RoomLampL settings: description=|
      | Bcm Buzzer output results.
      | 0 = None Buzzer
      | 1 = Turn signal Buzzer
      | 2 = Key Reminder Buzzer
      | 3 = Seat Belt Buzzer
      | 4 = Light Monitor Buzzer
  data AntitheftSta settings: description=|
      | 0 = Disarm Status
      | 1 = Arm Status
      | 2 = Wait for Rearm Status
      | 3 = Alarm Status
  events: eDrDoorLock local EITHER_EDGE_EVENT; eDrDoorUnlock local EITHER_EDGE_EVENT

== stateflow chart bcm/BCM/BCM/Tailgate/Chart ==
  settings: sampleTime=StepSize
  state TrunkRelease [parallel]
    settings: executionOrder=1
    state sStandBy
      en:TrunkRelease=0;
    state sDebounce
    state sUnlatch
      en:TrunkRelease=1;
    state sWaitForRelease
      en:TrunkRelease=0;
    (default) -> sStandBy
    sStandBy -> sDebounce : [TrunkHanSW==1]
    sDebounce -> (junction 1688) [order 1] : [after(20,tick)]
    (junction 1688) -> sUnlatch [order 1] : [!DrLockSta&&(PwrSta<=3||VehSpeed<5)]
    (junction 1688) -> sWaitForRelease [order 2]
    sDebounce -> sStandBy [order 2] : [TrunkHanSW==0]
    sUnlatch -> sWaitForRelease : [after(75,tick)]
    sWaitForRelease -> sStandBy : [TrunkHanSW==0]
  data: PwrSta input uint8 [0..4]; VehSpeed input [0..4047]; DrLockSta input boolean; TrunkRelease output boolean; TrunkHanSW input boolean
  data DrLockSta settings: description=Min=0, Max=2047, Engineering Unit = km/h, Offset=0 km/h, Resolution= 0.125 km/h per bit, >2047 = Invalid (bit 12 = 1)

== stateflow chart bcm/BCM/BCM/WasherWiper/Chart ==
  settings: sampleTime=StepSize
  state sWasher [parallel]
    settings: executionOrder=2  description=This state models the modes of a door sensor and implements logic to respond when that sensor is producing a signal.
    state sACCON
      state sFWasher
        note: 300 ms
        state sFrontWasher
          en:WasherControl=1;
        state sFrontWasher1
          en:WasherControl=1;
          FWasherCount=3;
        sFrontWasher -> sFrontWasher1 : [after(30,tick)]
      state sRWasher
        state sRearWasher
          en:WasherControl=2;
        state sRearWasher2
          en:WasherControl=2;
          RWasherCount=2;
        sRearWasher -> sRearWasher2 : [after(30,tick)]
      sFWasher -> (junction 1938) : [CSW_FWasSw_Sta!=1]
      sRWasher -> sFrontWasher [order 1] : [CSW_FWasSw_Sta==1]
      (junction 1938) -> (junction 1939) [order 1] : [CSW_RWasSW_Sta==1]
      (junction 1939) -> sRearWasher
    state sOFF
      en:WasherControl=0;
    (default) -> sWasher.sOFF
      settings: description=On the first sample call the door mode is set to active.
    sWasher.sOFF -> sFrontWasher [order 1] : [PwrSta>3&&CSW_FWasSw_Sta==1]
    (junction 1938) -> sWasher.sOFF [order 2]
    sACCON -> sWasher.sOFF : [PwrSta<=3]
    sWasher.sOFF -> sRearWasher [order 2] : [PwrSta>3&&CSW_RWasSW_Sta==1]
    sRWasher -> sWasher.sOFF [order 2] : [CSW_RWasSW_Sta!=1]
  state FrontWiper [parallel]
    settings: executionOrder=1
    state Wiping
      state sHIGHSPEED
        en:FWiperH=1;FWiperL=0;
      state sLOWSPEED
        en:FWiperH=0;FWiperL=1;
      FrontWiper.Wiping -> (junction 1869) [order 1]
      (junction 1869) -> sHIGHSPEED [order 1] : [CSW_FWipSw_Sta==3]
      (junction 1869) -> (junction 1870) [order 2]
      (junction 1870) -> (junction 1871) [order 1] : [CSW_FWipSw_Sta==1]
      (junction 1871) -> sLOWSPEED : [RLS_RainSnrWiperCmd==2 ||...
          |  RLS_RainSnrWiperCmd==3]
      (junction 1870) -> (junction 1873) [order 2]
      (junction 1873) -> sLOWSPEED [order 1] : [CSW_FWipSw_Sta==2]
      (junction 1873) -> (junction 1874) [order 2]
      (junction 1874) -> sLOWSPEED [order 1] : [CSW_FWasSw_Sta==2]
      (junction 1874) -> (junction 1875) [order 2]
      (junction 1875) -> (junction 1876) [order 1] : [FWasherCount>0]
      (junction 1876) -> sLOWSPEED [order 1] : [VINP_FWiperProtection_flg == 0]
      (junction 1876) -> (junction 1877) [order 2]
    state sOFF
      en:FWiperH=0;FWiperL=0;
    (default) -> FrontWiper.sOFF
    FrontWiper.sOFF -> (junction 1869) : [PwrSta>3]
    FrontWiper.Wiping -> FrontWiper.sOFF [order 1] : [PwrSta<=3]
    (junction 1875) -> FrontWiper.sOFF [order 2]
    (junction 1877) -> FrontWiper.sOFF : {FWasherCount = 0;}
  state RearWiper [parallel]
    settings: executionOrder=3
    state sOFF
      en:RWiper=0;
      RWasherCount=0;
    state Wiping
      state sON
        en:RWiper=1;
      note: 6 sec
      state sPark
      state sClean
      state sNotPark
        en:RWiper=0;
      sPark -> RearWiper.Wiping.sON : [after(600,tick)||RWasherCount>0||CSW_RWipIntSw_Sta==2]
      RearWiper.Wiping.sClean -> RearWiper.Wiping.sON : [RWiperAS==0]
      RearWiper.Wiping.sNotPark -> RearWiper.Wiping.sON [order 1] : [RWasherCount>0]
      RearWiper.Wiping.sON -> (junction 1912) : [RWiperAS==1]
      (junction 1913) -> RearWiper.Wiping.sClean [order 2] : {RWasherCount=RWasherCount-1;}
      (junction 1914) -> RearWiper.Wiping.sClean
      (junction 1912) -> (junction 1913) [order 1] : [RWasherCount>0]
      (junction 1913) -> (junction 1914) [order 1] : [WasherControl==2]
      (junction 1912) -> RearWiper.Wiping.sNotPark [order 2] : [CSW_RWipIntSw_Sta==1]
      RearWiper.Wiping.sNotPark -> sPark [order 2] : [RWiperAS==0]
    (default) -> RearWiper.sOFF
    RearWiper.sOFF -> (junction 1897) : [PwrSta>3]
    (junction 1897) -> RearWiper.Wiping.sON [order 2] : [CSW_RWipIntSw_Sta==1]
    (junction 1897) -> (junction 1898) [order 1]
    (junction 1898) -> RearWiper.Wiping.sON [order 2] : [CSW_RWipIntSw_Sta==2]
    (junction 1898) -> (junction 1899) [order 1]
    (junction 1899) -> RearWiper.Wiping.sON : [RWasherCount>0]
    RearWiper.Wiping -> RearWiper.sOFF [order 1] : [PwrSta <= 3]
    RearWiper.Wiping -> RearWiper.sOFF [order 2] : [VINP_RWiperProtection_flg == 1 && CSW_RWipIntSw_Sta==0]
    RearWiper.Wiping -> RearWiper.sOFF [order 3] : [CSW_RWipIntSw_Sta==0 && RWasherCount==0]
  state sFWasherWipingMode [parallel]
    settings: executionOrder=4
    state sOFF
      en:FWasherCount=0;
    state sON
      state sClean
        state sNotPark
          en:FWasherCount=FWasherCount-1;
        state sPark1
        (junction 1967) -> sFWasherWipingMode.sON.sClean.sNotPark [order 1] : [FWiperAS==1]
        sFWasherWipingMode.sON.sClean.sNotPark -> sPark1 : [FWiperAS==0]
        sPark1 -> sFWasherWipingMode.sON.sClean.sNotPark : [FWiperAS==1]
        (junction 1967) -> sPark1 [order 2]
      state ON
      ON -> (junction 1962) : [WasherControl!=1]
      (junction 1962) -> (junction 1967) [order 2]
      sFWasherWipingMode.sON.sClean -> ON [order 1] : [WasherControl==1]
    (default) -> sFWasherWipingMode.sOFF
    sFWasherWipingMode.sOFF -> ON : [PwrSta>3&&WasherControl==1]
    (junction 1962) -> sFWasherWipingMode.sOFF [order 1] : [FWasherCount == 0]
    sFWasherWipingMode.sON.sClean -> sFWasherWipingMode.sOFF [order 2] : [FWasherCount == 0]
    sFWasherWipingMode.sON -> sFWasherWipingMode.sOFF : [PwrSta <= 3]
  data: CSW_FWasSw_Sta input [0..3]; CSW_FWipSw_Sta input uint8 [0..7]; RLS_RainSnrWiperCmd input uint8 [0..7]; FWiperAS input boolean; FWiperL output boolean; FWiperH output boolean; FWasherCount local uint8; CSW_RWipIntSw_Sta input uint8 [0..3]; RWiper output boolean; RWiperAS input boolean; RWasherCount local uint8; CSW_RWasSW_Sta input; WasherControl output uint8; PwrSta input uint8 [0..5]; VINP_RWiperProtection_flg input; VINP_FWiperProtection_flg input

== matlab function bcm/BCM/BCM/AntiTheft/VIG_Decoder ==
  data: VINP_ReDoorLock_enum input; VIG_Cmd output
function VIG_Cmd = fcn(VINP_ReDoorLock_enum)
a=bitand(bitshift(VINP_ReDoorLock_enum,-12),15);
b=bitand(bitshift(VINP_ReDoorLock_enum,-8),15);
y=bitand(bitshift(VINP_ReDoorLock_enum,-4),15);
d=bitand(VINP_ReDoorLock_enum,15);
VIG_Cmd =bitxor(bitand(a,b),bitxor(y,d));

== stateflow chart bcm/BCM/BCM/AmbientLight/AmbientLight ==
  state OutputColor [parallel]
    settings: executionOrder=2
    (default) -> (junction 25) : {VBCM_AmbLightColor_enum=KBCM_AmbPreset_enum;}
    OutputColor -> (junction 25)
    (junction 25) -> (junction 28) [order 1] : [VINP_LINKtoDrive_flg]
    (junction 28) -> (junction 33) [order 1] : [VINP_IVIPWModeReq_enum==1]....
        | {VBCM_AmbLightColor_enum=KBCM_AmbRed_enum;}
    (junction 25) -> (junction 200) [order 2]
    (junction 28) -> (junction 35) [order 2]
    (junction 35) -> (junction 37) [order 1] : [VINP_IVIPWModeReq_enum==2]....
        | {VBCM_AmbLightColor_enum=KBCM_AmbGreen_enum;}
    (junction 35) -> (junction 39) [order 2]
    (junction 39) -> (junction 41) : {VBCM_AmbLightColor_enum=KBCM_AmbBlue_enum;}
    (junction 200) -> (junction 201) [order 1] : [VINP_AmbLightUser_enum==6]{VBCM_AmbLightColor_enum=VBCM_User6AmbLightColor_enum;}
    (junction 200) -> (junction 196) [order 2]
    (junction 196) -> (junction 197) [order 1] : [VINP_AmbLightUser_enum==5]{VBCM_AmbLightColor_enum=VBCM_User5AmbLightColor_enum;}
    (junction 196) -> (junction 30) [order 2]
    (junction 30) -> (junction 43) [order 1] : [VINP_AmbLightUser_enum==4]{VBCM_AmbLightColor_enum=VBCM_User4AmbLightColor_enum;}
    (junction 30) -> (junction 45) [order 2]
    (junction 45) -> (junction 47) [order 1] : [VINP_AmbLightUser_enum==3]{VBCM_AmbLightColor_enum=VBCM_User3AmbLightColor_enum;}
    (junction 45) -> (junction 49) [order 2]
    (junction 49) -> (junction 51) [order 1] : [VINP_AmbLightUser_enum==2]{VBCM_AmbLightColor_enum=VBCM_User2AmbLightColor_enum;}
    (junction 49) -> (junction 53) [order 2] : {VBCM_AmbLightColor_enum=VBCM_User1AmbLightColor_enum;}
  state ColorSettingReceiver [parallel]
    settings: executionOrder=1
    (default) -> (junction 5)
    ColorSettingReceiver -> (junction 3) : [hasChanged(VINP_AmbLightUserSet_enum)]
    (junction 3) -> (junction 5) [order 1] : [VINP_AmbLightUserSet_enum==1]....
        | {VBCM_User1AmbLightColor_enum=VINP_AmbLightColorSet_enum;}
    (junction 3) -> (junction 7) [order 2]
    (junction 7) -> (junction 9) [order 1] : [VINP_AmbLightUserSet_enum==2]....
        | {VBCM_User2AmbLightColor_enum=VINP_AmbLightColorSet_enum;}
    (junction 7) -> (junction 14) [order 2]
    (junction 14) -> (junction 16) [order 1] : [VINP_AmbLightUserSet_enum==3]....
        | {VBCM_User3AmbLightColor_enum=VINP_AmbLightColorSet_enum;}
    (junction 14) -> (junction 11) [order 2]
    (junction 11) -> (junction 20) [order 1] : [VINP_AmbLightUserSet_enum==4]....
        | {VBCM_User4AmbLightColor_enum=VINP_AmbLightColorSet_enum;}
    (junction 11) -> (junction 22) [order 2]
    (junction 22) -> (junction 184) [order 1] : [VINP_AmbLightUserSet_enum==5]....
        | {VBCM_User5AmbLightColor_enum=VINP_AmbLightColorSet_enum;}
    (junction 22) -> (junction 188) [order 2]
    (junction 188) -> (junction 185) : [VINP_AmbLightUserSet_enum==6]....
        | {VBCM_User6AmbLightColor_enum=VINP_AmbLightColorSet_enum;}
  state LampPower [parallel]
    settings: executionOrder=7
    state LampON
      state WaitForLampPwrON
        en:VBCM_LampPwr_flg=1;
      state LampPwrON
        en:VBCM_LampPwrReady_flg=true;
      (default) -> WaitForLampPwrON
      WaitForLampPwrON -> LampPwrON : after(5,tick)
    state OFF
      en:VBCM_LampPwr_flg=0;
      VBCM_LampPwrReady_flg=false;
    (default) -> OFF
    OFF -> LampON : [VBCM_WakeUp_flg==1||VPMM_PwrSta_enum>0]
    LampON -> OFF : [VBCM_WakeUp_flg==0&&VPMM_PwrSta_enum==0]
  state OutputBrightness [parallel]
    settings: executionOrder=5
    (default) -> (junction 92)
    OutputBrightness -> (junction 92) : [VBCM_LampPwrReady_flg]
    (junction 92) -> (junction 90) [order 1] : [VINP_IVINightModeSta_flg&&VBCM_PosLamp_flg||VPMM_PwrSta_enum<=3]....
        | {VBCM_IPAmbLightBrightness_enum=KBCM_ALMBrightnessDark_enum;
        | VBCM_DrAmbLightBrightness_enum=KBCM_ALMBrightnessDark_enum;}
    (junction 92) -> (junction 203) [order 2]
    (junction 203) -> (junction 324) [order 1] : [VINP_AmbLightUser_enum==6]....
        | {VBCM_IPAmbLightBrightness_enum=VBCM_User6IPAmbLightBrightness_enum;
        | VBCM_DrAmbLightBrightness_enum=VBCM_User6DrAmbLightBrightness_enum;}
    (junction 203) -> (junction 208) [order 2]
    (junction 324) -> (junction 347)
    (junction 208) -> (junction 347) [order 1] : [VINP_AmbLightUser_enum==5]....
        | {VBCM_IPAmbLightBrightness_enum=VBCM_User5IPAmbLightBrightness_enum;
        | VBCM_DrAmbLightBrightness_enum=VBCM_User5DrAmbLightBrightness_enum;}
    (junction 208) -> (junction 103) [order 2]
    (junction 347) -> (junction 360)
    (junction 103) -> (junction 360) [order 1] : [VINP_AmbLightUser_enum==4]....
        | {VBCM_IPAmbLightBrightness_enum=VBCM_User4IPAmbLightBrightness_enum;
        | VBCM_DrAmbLightBrightness_enum=VBCM_User4DrAmbLightBrightness_enum;}
    (junction 103) -> (junction 370) [order 2]
    (junction 360) -> (junction 373)
    (junction 370) -> (junction 373) [order 1] : [VINP_AmbLightUser_enum==3]....
        | {VBCM_IPAmbLightBrightness_enum=VBCM_User3IPAmbLightBrightness_enum;
        | VBCM_DrAmbLightBrightness_enum=VBCM_User3DrAmbLightBrightness_enum;}
    (junction 370) -> (junction 398) [order 2]
    (junction 373) -> (junction 409)
    (junction 398) -> (junction 409) [order 1] : [VINP_AmbLightUser_enum==2]....
        | {VBCM_IPAmbLightBrightness_enum=VBCM_User2IPAmbLightBrightness_enum;
        | VBCM_DrAmbLightBrightness_enum=VBCM_User2DrAmbLightBrightness_enum;}
    (junction 398) -> (junction 413) [order 2]
    (junction 409) -> (junction 415)
    (junction 413) -> (junction 415) : [VINP_AmbLightUser_enum==1]....
        | {VBCM_IPAmbLightBrightness_enum=VBCM_User1IPAmbLightBrightness_enum;
        | VBCM_DrAmbLightBrightness_enum=VBCM_User1DrAmbLightBrightness_enum;}
    (junction 415) -> (junction 176) [order 2]
    (junction 415) -> (junction 170) [order 1] : [!VINP_IVINightModeSta_flg&&VBCM_PosLamp_flg]....
        | {VBCM_IPAmbLightBrightness_enum=VBCM_IPAmbLightBrightness_enum/2;
        | VBCM_DrAmbLightBrightness_enum=VBCM_DrAmbLightBrightness_enum/2;}
  state WelcomeMode [parallel]
    settings: executionOrder=3
    state WaitForReady
    state StandBy
      en:VBCM_AmbLightBreath_flg=0;
    state Breath
      en:VBCM_AmbLightBreath_flg=1;
    WelcomeMode -> WaitForReady : [hasChanged(VINP_DrDoorSW_flg)&&VINP_DrDoorSW_flg]
    WaitForReady -> (junction 459) [order 2] : [after(KBCM_AmbBreathTOut_K,tick)]
    (junction 459) -> StandBy
    WaitForReady -> Breath [order 1] : [VPMM_PwrSta_enum>3]
    (default) -> StandBy
    Breath -> StandBy : [after(KBCM_AmbBreathT_K,tick)]
  state BrigthnessSettingReceiver [parallel]
    settings: executionOrder=4
    (default) -> (junction 74)
    BrigthnessSettingReceiver -> (junction 72) : [hasChanged(VINP_AmbLightUserSet_enum)]
    (junction 72) -> (junction 74) [order 1] : [VINP_AmbLightUserSet_enum==1]....
        | {VBCM_User1IPAmbLightBrightness_enum=VINP_IPAmbLightBrightnessSet_enum;
        | VBCM_User1DrAmbLightBrightness_enum=VINP_DrAmbLightBrightnessSet_enum;}
    (junction 72) -> (junction 77) [order 2]
    (junction 77) -> (junction 75) [order 1] : [VINP_AmbLightUserSet_enum==2]....
        | {VBCM_User2IPAmbLightBrightness_enum=VINP_IPAmbLightBrightnessSet_enum;
        | VBCM_User2DrAmbLightBrightness_enum=VINP_DrAmbLightBrightnessSet_enum;}
    (junction 77) -> (junction 79) [order 2]
    (junction 79) -> (junction 73) [order 1] : [VINP_AmbLightUserSet_enum==3]....
        | {VBCM_User3IPAmbLightBrightness_enum=VINP_IPAmbLightBrightnessSet_enum;
        | VBCM_User3DrAmbLightBrightness_enum=VINP_DrAmbLightBrightnessSet_enum;}
    (junction 79) -> (junction 80) [order 2]
    (junction 80) -> (junction 76) [order 1] : [VINP_AmbLightUserSet_enum==4]....
        | {VBCM_User4IPAmbLightBrightness_enum=VINP_IPAmbLightBrightnessSet_enum;
        | VBCM_User4DrAmbLightBrightness_enum=VINP_DrAmbLightBrightnessSet_enum;}
    (junction 80) -> (junction 78) [order 2]
    (junction 78) -> (junction 189) [order 1] : [VINP_AmbLightUserSet_enum==5]....
        | {VBCM_User5IPAmbLightBrightness_enum=VINP_IPAmbLightBrightnessSet_enum;
        | VBCM_User5DrAmbLightBrightness_enum=VINP_DrAmbLightBrightnessSet_enum;}
    (junction 78) -> (junction 194) [order 2]
    (junction 194) -> (junction 192) : [VINP_AmbLightUserSet_enum==6]....
        | {VBCM_User6IPAmbLightBrightness_enum=VINP_IPAmbLightBrightnessSet_enum;
        | VBCM_User6DrAmbLightBrightness_enum=VINP_DrAmbLightBrightnessSet_enum;}
  state ALM_Color_Brightness [parallel]
    settings: executionOrder=6
    (default) -> (junction 441)
    ALM_Color_Brightness -> (junction 441)
    (junction 441) -> (junction 462) : {VBCM_AmbLightBrightness1_enum=VBCM_IPAmbLightBrightness_enum;
        | VBCM_AmbLightBrightness2_enum=VBCM_DrAmbLightBrightness_enum;
        | VBCM_AmbLightBrightness3_enum=VBCM_DrAmbLightBrightness_enum;
        | VBCM_AmbLightColor1_enum=VBCM_AmbLightColor_enum;
        | VBCM_AmbLightColor2_enum=VBCM_AmbLightColor_enum;
        | VBCM_AmbLightColor3_enum=VBCM_AmbLightColor_enum;}
    (junction 462) -> (junction 444) [order 2] : {VBCM_AmbLightBreath1_flg=false;
        | VBCM_AmbLightBreath2_flg=false;
        | VBCM_AmbLightBreath3_flg=false;}
    (junction 462) -> (junction 464) [order 1] : [VBCM_IPAmbLightBrightness_enum>0||VBCM_DrAmbLightBrightness_enum>0]
        | {VBCM_AmbLightBreath1_flg=VBCM_AmbLightBreath_flg;
        | VBCM_AmbLightBreath2_flg=VBCM_AmbLightBreath_flg;
        | VBCM_AmbLightBreath3_flg=VBCM_AmbLightBreath_flg;}
  data: VINP_AmbLightColorSet_enum input; VINP_AmbLightUserSet_enum input; KBCM_ALMBrightnessDark_enum input; KBCM_AmbGreen_enum input; KBCM_AmbRed_enum input; VINP_LINKtoDrive_flg input; VINP_IVIPWModeReq_enum input; KBCM_AmbBlue_enum input; VINP_AmbLightUser_enum input; KBCM_AmbBreathT_K input; VINP_IVINightModeSta_flg input; VBCM_PosLamp_flg input; VINP_DrDoorSW_flg input; VBCM_User1AmbLightColor_enum output uint8 =0; VBCM_User4AmbLightColor_enum output uint8 =0; VBCM_User3AmbLightColor_enum output uint8 =0; VBCM_User2AmbLightColor_enum output uint8 =0; VPMM_PwrSta_enum input; VBCM_User1DrAmbLightBrightness_enum output uint8 =0; VBCM_User1IPAmbLightBrightness_enum output uint8 =0; VBCM_User2DrAmbLightBrightness_enum output uint8 =0; VBCM_User2IPAmbLightBrightness_enum output uint8 =0; VBCM_User3DrAmbLightBrightness_enum output uint8 =0; VBCM_User3IPAmbLightBrightness_enum output uint8 =0; VBCM_User4DrAmbLightBrightness_enum output uint8 =0; VBCM_User4IPAmbLightBrightness_enum output uint8 =0; VINP_IPAmbLightBrightnessSet_enum input; VINP_DrAmbLightBrightnessSet_enum input; VBCM_User5AmbLightColor_enum output uint8 =0; VBCM_User5DrAmbLightBrightness_enum output uint8 =0; VBCM_User5IPAmbLightBrightness_enum output uint8 =0; VBCM_User6AmbLightColor_enum output uint8 =0; VBCM_User6DrAmbLightBrightness_enum output uint8 =0; VBCM_User6IPAmbLightBrightness_enum output uint8 =0; VBCM_AmbLightBreath1_flg output boolean =0; VBCM_AmbLightBreath2_flg output boolean =0; VBCM_AmbLightBreath3_flg output boolean =0; VBCM_AmbLightBrightness1_enum output uint8 =0; VBCM_AmbLightBrightness2_enum output uint8 =0; VBCM_AmbLightBrightness3_enum output uint8 =0; VBCM_AmbLightColor1_enum output uint8 =0; VBCM_AmbLightColor2_enum output uint8 =0; VBCM_AmbLightColor3_enum output uint8 =0; KBCM_AmbPreset_enum input; VBCM_DrAmbLightBrightness_enum local double =0; VBCM_IPAmbLightBrightness_enum local double =0; VBCM_AmbLightBreath_flg local boolean =0; VBCM_AmbLightColor_enum local double =0; KBCM_AmbBreathTOut_K input; VBCM_LampPwr_flg output boolean; VBCM_WakeUp_flg input; VBCM_LampPwrReady_flg local boolean =0

== stateflow chart bcm/BCM/BCM/BCM_WAKE_MODULE/Chart ==
  state SleepReqJudge
    (default) -> (junction 3) : {
        |  VBCM_SleepReqLAST_flg = TRUE;
        |  VBCM_ConditionTimer_s = 0;
        |  }
    SleepReqJudge -> (junction 3)
    (junction 3) -> (junction 11) [order 2]
    (junction 3) -> (junction 7) [order 1] : [VBCM_SlpConditionMeet_flg]
    (junction 11) -> (junction 31) : {
        |   VBCM_SleepReq_flg = FALSE;
        |   VBCM_SleepReqLAST_flg = VBCM_SleepReq_flg;
        |   VBCM_ConditionTimer_s = 0;
        | }
    (junction 7) -> (junction 17) [order 2]
    (junction 7) -> (junction 26) [order 1] : [VBCM_SleepReqLAST_flg]
    (junction 17) -> (junction 19) : {VBCM_ConditionTimer_s += task_time_s;}
    (junction 19) -> (junction 31) [order 2]
    (junction 19) -> (junction 24) [order 1] : [VBCM_ConditionTimer_s >= KBCM_SlpDebounceTime_s]
    (junction 31) -> (junction 13)
    (junction 24) -> (junction 26)
    (junction 26) -> (junction 29) : {
        |  VBCM_SleepReq_flg = TRUE;
        |  VBCM_SleepReqLAST_flg = VBCM_SleepReq_flg;
        |  VBCM_ConditionTimer_s = 0;
        | }
    (junction 29) -> (junction 13)
  (default) -> SleepReqJudge
  data: TRUE parameter; VBCM_SleepReq_flg output boolean; VBCM_ConditionTimer_s local single; VBCM_SlpConditionMeet_flg input; FALSE parameter; VBCM_SleepReqLAST_flg local boolean; task_time_s input; KBCM_SlpDebounceTime_s input
